simulink model "BP_RBFNN_Sim"  (R2022a)
settings: Solver=ode4  StartTime=0.0  StopTime=15  FixedStep=0.001  RelTol=1e-3
libraries: simulink x1
settings Model: Creator=Userx  LastModifiedBy=Userx

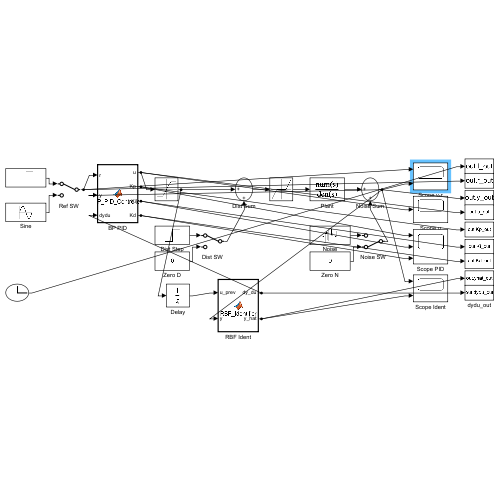
[thumbnail: Simulink's stored preview of the top-level diagram]
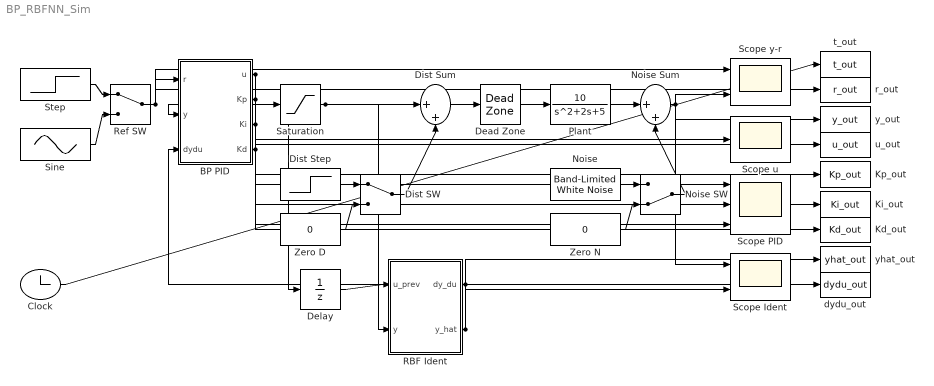
== system BP_RBFNN_Sim ==
  BP PID : MATLAB Function  TreatAsAtomicUnit=on  SystemSampleTime=0.001
  Clock : Clock
  Dead Zone : DeadZone  LowerValue=-0.3  UpperValue=0.3
  Delay : UnitDelay  SampleTime=0.001  HasFrameUpgradeWarning=on
  Dist SW : ManualSwitch
  Dist Step : Step  Time=8  After=1.5  SampleTime=0
  Dist Sum : Sum  Inputs=|++
  Kd_out : ToWorkspace  VariableName=Kd_out  SaveFormat=Timeseries  SampleTime=-1
  Ki_out : ToWorkspace  VariableName=Ki_out  SaveFormat=Timeseries  SampleTime=-1
  Kp_out : ToWorkspace  VariableName=Kp_out  SaveFormat=Timeseries  SampleTime=-1
  Noise : simulink/Sources/Band-Limited White Noise  Cov=0.0001  Ts=0.001  seed=23341
  Noise SW : ManualSwitch  CurrentSetting=0
  Noise Sum : Sum  Inputs=|++
  Plant : TransferFcn  Numerator=[10]  Denominator=[1 2 5]
  RBF Ident : MATLAB Function  TreatAsAtomicUnit=on  SystemSampleTime=0.001
  Ref SW : ManualSwitch
  Saturation : Saturate  UpperLimit=10  LowerLimit=-10
  Scope Ident : Scope  NumInputPorts=2
  Scope PID : Scope  NumInputPorts=3
  Scope u : Scope
  Scope y-r : Scope  NumInputPorts=2
  Sine : Sin  Frequency=0.5  SampleTime=0
  Step : Step  Time=0.5  SampleTime=0
  Zero D : Constant  Value=0
  Zero N : Constant  Value=0
  dydu_out : ToWorkspace  VariableName=dydu_out  SaveFormat=Timeseries  SampleTime=-1
  r_out : ToWorkspace  VariableName=r_out  SaveFormat=Timeseries  SampleTime=-1
  t_out : ToWorkspace  VariableName=t_out  SaveFormat=Timeseries  SampleTime=-1
  u_out : ToWorkspace  VariableName=u_out  SaveFormat=Timeseries  SampleTime=-1
  y_out : ToWorkspace  VariableName=y_out  SaveFormat=Timeseries  SampleTime=-1
  yhat_out : ToWorkspace  VariableName=yhat_out  SaveFormat=Timeseries  SampleTime=-1
  wires:
  Step/1 -> Ref SW/1
  Sine/1 -> Ref SW/2
  Ref SW/1 -> BP PID/1(r), Scope y-r/1, r_out/1
  BP PID/1(u) -> Saturation/1, Scope u/1, u_out/1
  Saturation/1 -> Dist Sum/1, Delay/1
  Dist Step/1 -> Dist SW/1
  Zero D/1 -> Dist SW/2
  Dist SW/1 -> Dist Sum/2
  Dist Sum/1 -> Dead Zone/1
  Dead Zone/1 -> Plant/1
  Plant/1 -> Noise Sum/1
  Noise/1 -> Noise SW/1
  Zero N/1 -> Noise SW/2
  Noise SW/1 -> Noise Sum/2
  Noise Sum/1 -> BP PID/2(y), RBF Ident/2(y), Scope y-r/2, Scope Ident/1, y_out/1
  Delay/1 -> RBF Ident/1(u_prev)
  RBF Ident/1(dy_du) -> BP PID/3(dydu), dydu_out/1
  BP PID/2(Kp) -> Scope PID/1, Kp_out/1
  BP PID/3(Ki) -> Scope PID/2, Ki_out/1
  BP PID/4(Kd) -> Scope PID/3, Kd_out/1
  RBF Ident/2(y_hat) -> Scope Ident/2, yhat_out/1
  Clock/1 -> t_out/1

== matlab function BP_RBFNN_Sim/RBF Ident ==
  data: u_prev input; dy_du output; y input; y_hat output
function [dy_du, y_hat] = RBF_Identifier(u_prev, y)
% =========================================================================
% RBF Neural Network Online System Identifier
% =========================================================================
% 网络结构: 4输入 → M个RBF节点(高斯核) → 1输出
%
% 输入:
%   u_prev - u(k-1), 经Unit Delay的控制量 (避免代数环)
%   y      - y(k), 被控对象当前输出
%
% 输出:
%   dy_du  - 雅可比 ∂ŷ/∂u(k-1), 供BP-PID反传使用
%   y_hat  - RBF网络预测输出, 用于监控辨识精度
%
% 输入向量: x(k) = [y(k-1), y(k-2), u(k-1), u(k-2)]
%   u(k-1)来自外部端口, u(k-2)由persistent延迟寄存器提供
%   y(k-1), y(k-2)同理
%
% 在线学习: 每步基于辨识误差e_id = y - ŷ的梯度下降
% =========================================================================

%% ===== 超参数 =====
M       = 10;     % RBF隐层节点数
n       = 4;      % 输入维度 [y(k-1), y(k-2), u(k-1), u(k-2)]
eta_w   = 0.35;   % 输出权值 W 学习率
eta_c   = 0.06;   % 中心 C 学习率
eta_s   = 0.06;   % 宽度 σ 学习率
mu_w    = 0.05;   % W 动量系数
mu_c    = 0.03;   % C 动量系数
mu_s    = 0.03;   % σ 动量系数
sig_min = 0.01;   % σ 下界 (防止除零和数值不稳定)

%% ===== 持久变量 =====
persistent W C Sigma
persistent dW_prev dC_prev dSig_prev
persistent y1 y2 u2          % 延迟寄存器
persistent init_flag

%% ===== 初始化 =====
if isempty(init_flag)
    % W: 小随机值, 正负各半
    W = 0.15 * randn(1, M);
    % C: 在输入空间均匀分布 + 随机扰动
    C = repmat(linspace(-1.2, 1.2, M)', 1, n) + 0.1 * randn(M, n);
    % Sigma: 初始宽度覆盖输入空间
    Sigma = 1.5 * ones(M, 1);
    % 动量项初始化为零
    dW_prev   = zeros(1, M);
    dC_prev   = zeros(M, n);
    dSig_prev = zeros(M, 1);
    % 延迟寄存器
    y1 = 0;  y2 = 0;  u2 = 0;
    init_flag = true;
end

%% ===== 构造输入向量 =====
% x = [y(k-1); y(k-2); u(k-1); u(k-2)]
x = [y1; y2; double(u_prev); u2];   % 4×1

%% ===== 前向传播 =====
% D: M×n, 每行是输入向量到第i个中心的欧氏距离分量
D = bsxfun(@minus, x', C);              % M×n  (x' is 1×n, C is M×n)
dist2 = sum(D .^ 2, 2);                 % M×1  平方欧氏距离
H = exp(-dist2 ./ (2 * Sigma .^ 2));    % M×1  高斯核激活值
y_hat = W * H;                          % 标量  网络预测输出

%% ===== 辨识误差 =====
e_id = double(y) - y_hat;

%% ===== 梯度计算 =====
% ∂E/∂W = -e_id * H^T,  E=0.5*e_id^2
grad_W = -e_id * H';                    % 1×M

% ∂E/∂C 和 ∂E/∂σ 的公共缩放因子
scale = (W .* H') ./ (Sigma .^ 2)';     % 1×M

% ∂E/∂C: 利用bsxfun逐元素乘
grad_C = -e_id * bsxfun(@times, D, scale');    % M×n

% ∂E/∂σ = -e_id * W' .* H .* dist2 ./ σ^3
grad_S = -e_id * (W' .* H .* dist2 ./ (Sigma .^ 3));   % M×1

%% ===== 带动量的参数更新 =====
dW   = -eta_w * grad_W + mu_w * dW_prev;
dC   = -eta_c * grad_C + mu_c * dC_prev;
dS   = -eta_s * grad_S + mu_s * dSig_prev;

W     = W + dW;
C     = C + dC;
Sigma = max(Sigma + dS, sig_min);       % 保证σ>0

% 保存动量项
dW_prev   = dW;
dC_prev   = dC;
dSig_prev = dS;

%% ===== 计算雅可比 ∂ŷ/∂u(k-1) =====
% u(k-1) 在输入向量 x 中是第3个分量, 对应 D 的第3列
% ∂ŷ/∂u = Σ W_i * H_i * (-(u - c_{i,u}) / σ_i^2)
dy_du = sum(W' .* H .* (-D(:,3) ./ Sigma .^ 2));

% 雅可比下限: 避免梯度为零导致BP-PID停止学习
if abs(dy_du) < 1e-4
    dy_du = sign(dy_du + eps) * 1e-4;
end

%% ===== 更新延迟寄存器 =====
y2 = y1;
y1 = double(y);
u2 = double(u_prev);     % 当前u(k-1)在下一步变为u(k-2)

end

== matlab function BP_RBFNN_Sim/BP PID ==
  data: r input; u output; y input; dydu input; Kp output; Ki output; Kd output
function [u, Kp, Ki, Kd] = BP_PID_Controller(r, y, dydu)
% =========================================================================
% BP Neural Network Self-Tuning PID Controller
% =========================================================================
% 网络结构: 3输入 → M隐层(tanh) → 3输出(sigmoid→映射到PID参数范围)
%
% 输入:
%   r    - 设定值 (reference)
%   y    - 被控对象输出 (plant output, 含噪声的测量值)
%   dydu - RBF辨识器提供的雅可比 ∂y/∂u
%
% 输出:
%   u    - 控制量 (增量式PID累加, 含限幅)
%   Kp,Ki,Kd - 实时PID参数 (用于在线监控)
%
% 在线学习: 每步基于梯度链 ∂E/∂W 更新网络权值
%   E = 0.5*(r-y)^2 → BP反传 → W ← W - lr*∂E/∂W
% =========================================================================

%% ===== 超参数 =====
M        = 6;       % 隐层神经元数
lr       = 0.015;   % 学习率
momentum = 0.05;    % 动量系数
Ts       = 0.001;   % 采样周期 (需与Simulink固定步长一致)
grad_clip = 1.0;    % 梯度裁剪阈值

% PID参数映射范围 (sigmoid输出映射到此区间)
Kp_min = 0;    Kp_max = 50;
Ki_min = 0;    Ki_max = 20;
Kd_min = 0;    Kd_max = 10;

% 控制量限幅
u_min = -10;
u_max =  10;

%% ===== 持久变量 =====
persistent W1 W2 b1 b2               % 网络权值与偏置
persistent dW1_prev dW2_prev         % 上一步权值更新量(动量用)
persistent db1_prev db2_prev
persistent e1 e2 u_prev sum_e        % 历史状态
persistent is_init

nin  = 3;   % [e, de, sum_e]
nout = 3;   % [Kp, Ki, Kd]

%% ===== 初始化 =====
if isempty(is_init)
    W1 = (rand(M, nin)  - 0.5) * 2 * sqrt(2/nin);   % He初始化, 配合tanh
    W2 = (rand(nout, M) - 0.5) * 2 * sqrt(2/M);
    b1 = zeros(M, 1);
    b2 = zeros(nout, 1);

    dW1_prev = zeros(M, nin);
    dW2_prev = zeros(nout, M);
    db1_prev = zeros(M, 1);
    db2_prev = zeros(nout, 1);

    e1     = 0;
    e2     = 0;
    u_prev = 0;
    sum_e  = 0;
    is_init = true;
end

%% ===== 误差信号 =====
e    = r - y;
de   = e - e1;
d2e  = e - 2*e1 + e2;
sum_e = sum_e + e * Ts;

%% ===== 前向传播 =====
x = [e; de; sum_e];                     % 3×1 输入向量

net_h = W1 * x + b1;                    % M×1
h     = tanh(net_h);                    % 隐层激活

net_o = W2 * h + b2;                    % 3×1
o     = 1 ./ (1 + exp(-net_o));         % 输出层sigmoid, o∈(0,1)

% 映射到物理PID参数
Kp = Kp_min + (Kp_max - Kp_min) * o(1);
Ki = Ki_min + (Ki_max - Ki_min) * o(2);
Kd = Kd_min + (Kd_max - Kd_min) * o(3);

%% ===== 增量式PID =====
delta_u = Kp * de + Ki * e + Kd * d2e;
u = u_prev + delta_u;
u = max(u_min, min(u_max, u));

%% ===== 在线反向传播 =====
% 性能指标: E = 0.5*e^2

% dE/du = dE/dy * dy/du = -e * dydu
dE_du = -e * dydu;

% du/dKj: 增量PID对各参数的偏导数
%   ∂u/∂Kp ≈ de, ∂u/∂Ki ≈ e, ∂u/∂Kd ≈ d2e
du_dK = [de; e; d2e];

% dKj/doj: 线性映射的缩放因子
scale_K = [Kp_max - Kp_min; Ki_max - Ki_min; Kd_max - Kd_min];

% doj/dnet_oj: sigmoid导数
dsig = o .* (1 - o);    % sigmoid'(x) = sigmoid(x)*(1-sigmoid(x))

% 输出层误差信号 δo = dE/du * du/dK * dK/do * do/dnet_o
delta_o = dE_du * (du_dK .* scale_K .* dsig);

% 隐层误差信号 δh = W2'*δo .* tanh'(net_h)
delta_h = (W2' * delta_o) .* (1 - h.^2);   % tanh'(x) = 1 - tanh^2(x)

% 梯度裁剪
delta_o = max(-grad_clip, min(grad_clip, delta_o));
delta_h = max(-grad_clip, min(grad_clip, delta_h));

% 计算梯度
grad_W2 = delta_o * h';                    % 3×M
grad_b2 = delta_o;                         % 3×1
grad_W1 = delta_h * x';                    % M×3
grad_b1 = delta_h;                         % M×1

% 带动量的权值更新
dW2 = lr * grad_W2 + momentum * dW2_prev;
db2 = lr * grad_b2 + momentum * db2_prev;
dW1 = lr * grad_W1 + momentum * dW1_prev;
db1 = lr * grad_b1 + momentum * db1_prev;

W2 = W2 - dW2;
b2 = b2 - db2;
W1 = W1 - dW1;
b1 = b1 - db1;

% 保存动量项
dW2_prev = dW2;
db2_prev = db2;
dW1_prev = dW1;
db1_prev = db1;

%% ===== 更新历史状态 =====
e2     = e1;
e1     = e;
u_prev = u;

end
